simulink model "untitled"  (R2016a)
settings: Solver=VariableStepAuto  StartTime=0.0  StopTime=100  RelTol=1e-3
libraries: simulink x1
settings Model: Creator=NAD  LastModifiedBy=NAD

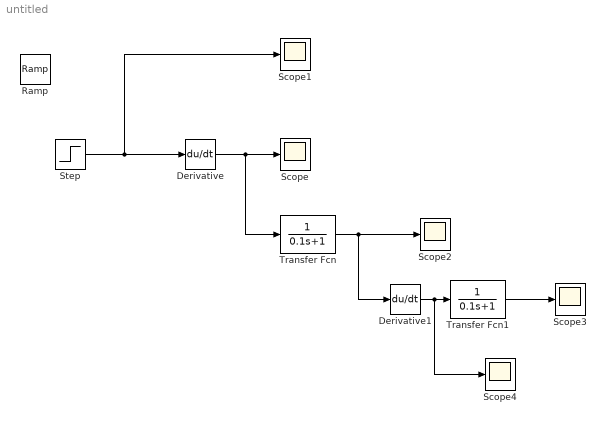
== system untitled ==
  Derivative : Derivative
  Derivative1 : Derivative
  Ramp : simulink/Sources/Ramp  slope=1  start=0  X0=0
  Scope{,1..4} (5 alike) : Scope
  Step : Step  SampleTime=0
  Transfer Fcn : TransferFcn  Denominator=[0.1 1 ]
  Transfer Fcn1 : TransferFcn  Denominator=[0.1 1 ]
  wires:
  Derivative/1 -> Transfer Fcn/1, Scope/1
  Transfer Fcn/1 -> Derivative1/1, Scope2/1
  Step/1 -> Derivative/1, Scope1/1
  Derivative1/1 -> Scope4/1, Transfer Fcn1/1
  Transfer Fcn1/1 -> Scope3/1
